simulink model "threshold_estimator"  (R2021a)
settings: Solver=FixedStepDiscrete  StartTime=0.0  StopTime=7.93555  RelTol=1e-3
undefined symbols (not defined in the file): lambda2
settings Model: DataTypeOverride=Off  Creator=Bhea Vasquez  LastModifiedBy=Bhea Vasquez
settings OptimizationCC: BlockReduction=off  ConditionallyExecuteInputs=off  DefaultParameterBehavior=Inlined
settings DebuggingCC: AlgebraicLoopMsg=error  SingleTaskRateTransMsg=error
settings HardwareCC: ProdBitPerPointer=32  ProdBitPerSizeT=32  ProdBitPerPtrDiffT=32  ProdLargestAtomicFloat=None  ProdIntDivRoundTo=Undefined  ProdEndianess=Unspecified  ProdWordSize=32  ProdHWDeviceType=ASIC/FPGA->ASIC/FPGA  TargetBitPerPointer=64  TargetBitPerSizeT=64  TargetBitPerPtrDiffT=64  TargetLongLongMode=on  TargetIntDivRoundTo=Zero  TargetEndianess=LittleEndian  TargetWordSize=64  TargetHWDeviceType=Custom Processor->MATLAB Host Computer  ProdEqTarget=off

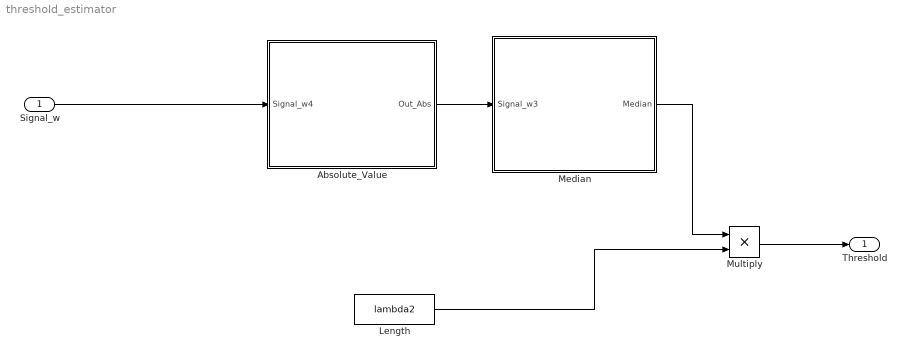
== system threshold_estimator ==
  Signal_w : Inport  OutDataTypeStr=fixdt(1,16,12)
  Absolute_Value : Subsystem
  Length : Constant  Value=lambda2  OutDataTypeStr=fixdt(1,16,12)  SampleTime=-1
  Median : Subsystem
  Multiply : Product  OutDataTypeStr=fixdt(1,16,12)  LockScale=on
  Threshold : Outport  OutDataTypeStr=fixdt(1,16,12)  VectorParamsAs1DForOutWhenUnconnected=off
  wires:
  Absolute_Value/1(Out_Abs) -> Median/1(Signal_w3)
  Signal_w/1 -> Absolute_Value/1(Signal_w4)
  Length/1 -> Multiply/2
  Multiply/1 -> Threshold/1
  Median/1(Median) -> Multiply/1

== system threshold_estimator/Absolute_Value ==
  Signal_w4 : Inport  OutDataTypeStr=fixdt(1,16,12)
  Absolute_Switch : Switch  Threshold=1  OutDataTypeStr=fixdt(1,16,12)
  Constant295 : Constant  Value=0  OutDataTypeStr=fixdt(1,16,12)  SampleTime=-1
  Gain2 : Gain  Gain=-1  ParamDataTypeStr=fixdt(1,16,12)  OutMin=-1  OutMax=-0.99  OutDataTypeStr=fixdt(1,16,12)
  Relational Operator2 : RelationalOperator  Operator=<  OutDataTypeStr=fixdt(1,16,12)  RndMeth=Simplest
  Out_Abs : Outport  OutDataTypeStr=fixdt(1,16,12)  VectorParamsAs1DForOutWhenUnconnected=off
  wires:
  Absolute_Switch/1 -> Out_Abs/1
  Relational Operator2/1 -> Absolute_Switch/2
  Gain2/1 -> Absolute_Switch/1
  Signal_w4/1 -> Absolute_Switch/3, Relational Operator2/1, Gain2/1
  Constant295/1 -> Relational Operator2/2

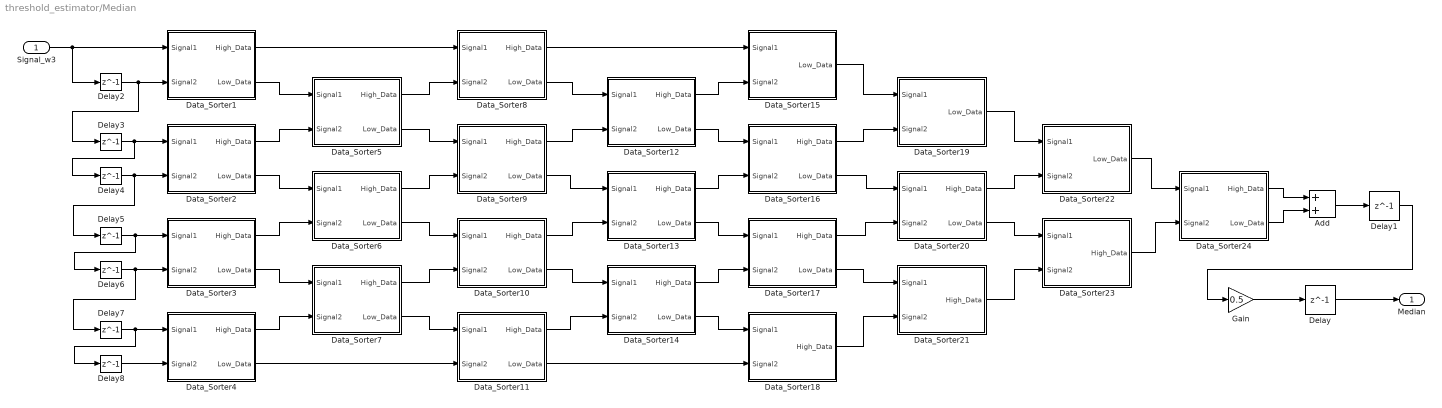
== system threshold_estimator/Median ==
  Signal_w3 : Inport  OutDataTypeStr=fixdt(1,16,12)
  Add : Sum  AccumDataTypeStr=fixdt(1,16,12)  OutDataTypeStr=fixdt(1,16,12)  LockScale=on
  Data_Sorter1 : Subsystem
  Data_Sorter10 : Subsystem
  Data_Sorter11 : Subsystem
  Data_Sorter12 : Subsystem
  Data_Sorter13 : Subsystem
  Data_Sorter14 : Subsystem
  Data_Sorter15 : Subsystem
  Data_Sorter16 : Subsystem
  Data_Sorter17 : Subsystem
  Data_Sorter18 : Subsystem
  Data_Sorter19 : Subsystem
  Data_Sorter2 : Subsystem
  Data_Sorter20 : Subsystem
  Data_Sorter21 : Subsystem
  Data_Sorter22 : Subsystem
  Data_Sorter23 : Subsystem
  Data_Sorter24 : Subsystem
  Data_Sorter3 : Subsystem
  Data_Sorter4 : Subsystem
  Data_Sorter5 : Subsystem
  Data_Sorter6 : Subsystem
  Data_Sorter7 : Subsystem
  Data_Sorter8 : Subsystem
  Data_Sorter9 : Subsystem
  Delay{,1..8} (9 alike) : Delay  DelayLength=1
  Gain : Gain  Gain=0.5  ParamDataTypeStr=fixdt(1,16,12)  OutMin=0.499  OutMax=0.5  OutDataTypeStr=fixdt(1,16,12)
  Median : Outport  OutDataTypeStr=fixdt(1,16,12)  VectorParamsAs1DForOutWhenUnconnected=off
  wires:
  Data_Sorter4/1(High_Data) -> Data_Sorter7/2(Signal2)
  Delay3/1 -> Delay4/1, Data_Sorter2/1(Signal1)
  Signal_w3/1 -> Data_Sorter1/1(Signal1), Delay2/1
  Data_Sorter10/1(High_Data) -> Data_Sorter13/2(Signal2)
  Data_Sorter23/1(High_Data) -> Data_Sorter24/2(Signal2)
  Data_Sorter12/2(Low_Data) -> Data_Sorter16/1(Signal1)
  Delay2/1 -> Delay3/1, Data_Sorter1/2(Signal2)
  Data_Sorter5/1(High_Data) -> Data_Sorter8/2(Signal2)
  Delay/1 -> Median/1
  Data_Sorter15/1(Low_Data) -> Data_Sorter19/1(Signal1)
  Add/1 -> Delay1/1
  Data_Sorter7/2(Low_Data) -> Data_Sorter11/1(Signal1)
  Data_Sorter24/1(High_Data) -> Add/1
  Data_Sorter1/2(Low_Data) -> Data_Sorter5/1(Signal1)
  Data_Sorter3/1(High_Data) -> Data_Sorter6/2(Signal2)
  Data_Sorter22/1(Low_Data) -> Data_Sorter24/1(Signal1)
  Data_Sorter2/1(High_Data) -> Data_Sorter5/2(Signal2)
  Data_Sorter10/2(Low_Data) -> Data_Sorter14/1(Signal1)
  Delay1/1 -> Gain/1
  Data_Sorter17/2(Low_Data) -> Data_Sorter21/1(Signal1)
  Data_Sorter21/1(High_Data) -> Data_Sorter23/2(Signal2)
  Data_Sorter7/1(High_Data) -> Data_Sorter10/2(Signal2)
  Delay4/1 -> Delay5/1, Data_Sorter2/2(Signal2)
  Data_Sorter16/1(High_Data) -> Data_Sorter19/2(Signal2)
  Data_Sorter20/1(High_Data) -> Data_Sorter22/2(Signal2)
  Data_Sorter16/2(Low_Data) -> Data_Sorter20/1(Signal1)
  Data_Sorter3/2(Low_Data) -> Data_Sorter7/1(Signal1)
  Data_Sorter2/2(Low_Data) -> Data_Sorter6/1(Signal1)
  Data_Sorter6/2(Low_Data) -> Data_Sorter10/1(Signal1)
  Data_Sorter19/1(Low_Data) -> Data_Sorter22/1(Signal1)
  Data_Sorter12/1(High_Data) -> Data_Sorter15/2(Signal2)
  Data_Sorter5/2(Low_Data) -> Data_Sorter9/1(Signal1)
  Data_Sorter24/2(Low_Data) -> Add/2
  Data_Sorter17/1(High_Data) -> Data_Sorter20/2(Signal2)
  Data_Sorter13/1(High_Data) -> Data_Sorter16/2(Signal2)
  Data_Sorter11/1(High_Data) -> Data_Sorter14/2(Signal2)
  Delay8/1 -> Data_Sorter4/2(Signal2)
  Data_Sorter8/2(Low_Data) -> Data_Sorter12/1(Signal1)
  Delay6/1 -> Delay7/1, Data_Sorter3/2(Signal2)
  Data_Sorter9/2(Low_Data) -> Data_Sorter13/1(Signal1)
  Data_Sorter4/2(Low_Data) -> Data_Sorter11/2(Signal2)
  Data_Sorter9/1(High_Data) -> Data_Sorter12/2(Signal2)
  Data_Sorter14/2(Low_Data) -> Data_Sorter18/1(Signal1)
  Delay5/1 -> Delay6/1, Data_Sorter3/1(Signal1)
  Delay7/1 -> Delay8/1, Data_Sorter4/1(Signal1)
  Data_Sorter1/1(High_Data) -> Data_Sorter8/1(Signal1)
  Data_Sorter8/1(High_Data) -> Data_Sorter15/1(Signal1)
  Data_Sorter14/1(High_Data) -> Data_Sorter17/2(Signal2)
  Data_Sorter6/1(High_Data) -> Data_Sorter9/2(Signal2)
  Data_Sorter20/2(Low_Data) -> Data_Sorter23/1(Signal1)
  Data_Sorter11/2(Low_Data) -> Data_Sorter18/2(Signal2)
  Data_Sorter13/2(Low_Data) -> Data_Sorter17/1(Signal1)
  Gain/1 -> Delay/1
  Data_Sorter18/1(High_Data) -> Data_Sorter21/2(Signal2)

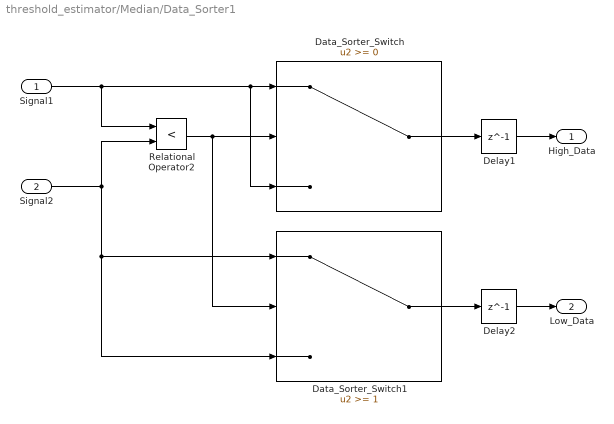
== system threshold_estimator/Median/Data_Sorter1 ==
  Signal1 : Inport  OutDataTypeStr=fixdt(1,16,12)
  Signal2 : Inport  Port=2  OutDataTypeStr=fixdt(1,16,12)
  Data_Sorter_Switch : Switch  OutDataTypeStr=fixdt(1,16,12)
  Data_Sorter_Switch1 : Switch  Threshold=1  OutDataTypeStr=fixdt(1,16,12)
  Delay1 : Delay  DelayLength=1
  Delay2 : Delay  DelayLength=1
  Relational Operator2 : RelationalOperator  Operator=<  OutDataTypeStr=fixdt(1,16,12)  RndMeth=Simplest
  High_Data : Outport  OutDataTypeStr=fixdt(1,16,12)  VectorParamsAs1DForOutWhenUnconnected=off
  Low_Data : Outport  Port=2  OutDataTypeStr=fixdt(1,16,12)  VectorParamsAs1DForOutWhenUnconnected=off
  wires:
  Signal1/1 -> Data_Sorter_Switch/3, Data_Sorter_Switch/1, Relational Operator2/1
  Relational Operator2/1 -> Data_Sorter_Switch1/2, Data_Sorter_Switch/2
  Signal2/1 -> Data_Sorter_Switch1/1, Data_Sorter_Switch1/3, Relational Operator2/2
  Data_Sorter_Switch1/1 -> Delay2/1
  Delay2/1 -> Low_Data/1
  Data_Sorter_Switch/1 -> Delay1/1
  Delay1/1 -> High_Data/1

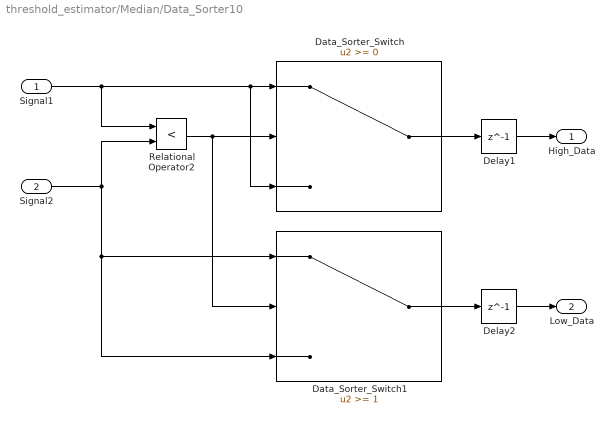
== system threshold_estimator/Median/Data_Sorter10 ==
  Signal1 : Inport  OutDataTypeStr=fixdt(1,16,12)
  Signal2 : Inport  Port=2  OutDataTypeStr=fixdt(1,16,12)
  Data_Sorter_Switch : Switch  OutDataTypeStr=fixdt(1,16,12)
  Data_Sorter_Switch1 : Switch  Threshold=1  OutDataTypeStr=fixdt(1,16,12)
  Delay1 : Delay  DelayLength=1
  Delay2 : Delay  DelayLength=1
  Relational Operator2 : RelationalOperator  Operator=<  OutDataTypeStr=fixdt(1,16,12)  RndMeth=Simplest
  High_Data : Outport  OutDataTypeStr=fixdt(1,16,12)  VectorParamsAs1DForOutWhenUnconnected=off
  Low_Data : Outport  Port=2  OutDataTypeStr=fixdt(1,16,12)  VectorParamsAs1DForOutWhenUnconnected=off
  wires:
  Signal1/1 -> Data_Sorter_Switch/3, Data_Sorter_Switch/1, Relational Operator2/1
  Relational Operator2/1 -> Data_Sorter_Switch1/2, Data_Sorter_Switch/2
  Signal2/1 -> Data_Sorter_Switch1/1, Data_Sorter_Switch1/3, Relational Operator2/2
  Data_Sorter_Switch1/1 -> Delay2/1
  Delay2/1 -> Low_Data/1
  Data_Sorter_Switch/1 -> Delay1/1
  Delay1/1 -> High_Data/1

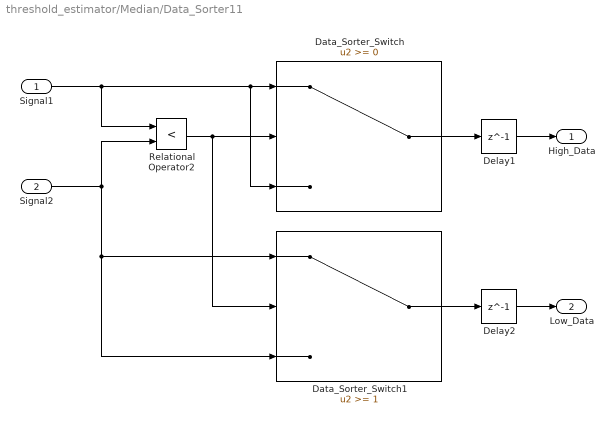
== system threshold_estimator/Median/Data_Sorter11 ==
  Signal1 : Inport  OutDataTypeStr=fixdt(1,16,12)
  Signal2 : Inport  Port=2  OutDataTypeStr=fixdt(1,16,12)
  Data_Sorter_Switch : Switch  OutDataTypeStr=fixdt(1,16,12)
  Data_Sorter_Switch1 : Switch  Threshold=1  OutDataTypeStr=fixdt(1,16,12)
  Delay1 : Delay  DelayLength=1
  Delay2 : Delay  DelayLength=1
  Relational Operator2 : RelationalOperator  Operator=<  OutDataTypeStr=fixdt(1,16,12)  RndMeth=Simplest
  High_Data : Outport  OutDataTypeStr=fixdt(1,16,12)  VectorParamsAs1DForOutWhenUnconnected=off
  Low_Data : Outport  Port=2  OutDataTypeStr=fixdt(1,16,12)  VectorParamsAs1DForOutWhenUnconnected=off
  wires:
  Signal1/1 -> Data_Sorter_Switch/3, Data_Sorter_Switch/1, Relational Operator2/1
  Relational Operator2/1 -> Data_Sorter_Switch1/2, Data_Sorter_Switch/2
  Signal2/1 -> Data_Sorter_Switch1/1, Data_Sorter_Switch1/3, Relational Operator2/2
  Data_Sorter_Switch1/1 -> Delay2/1
  Delay2/1 -> Low_Data/1
  Data_Sorter_Switch/1 -> Delay1/1
  Delay1/1 -> High_Data/1

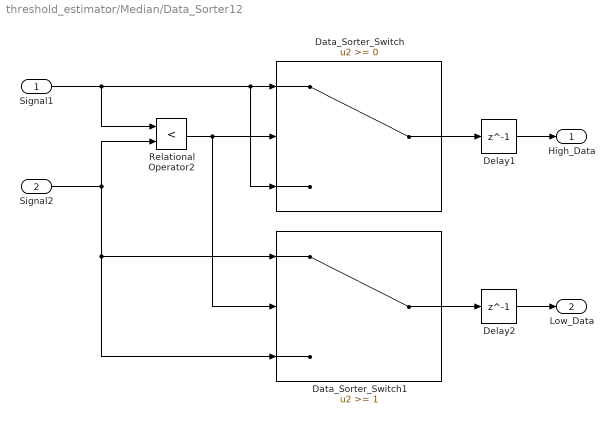
== system threshold_estimator/Median/Data_Sorter12 ==
  Signal1 : Inport  OutDataTypeStr=fixdt(1,16,12)
  Signal2 : Inport  Port=2  OutDataTypeStr=fixdt(1,16,12)
  Data_Sorter_Switch : Switch  OutDataTypeStr=fixdt(1,16,12)
  Data_Sorter_Switch1 : Switch  Threshold=1  OutDataTypeStr=fixdt(1,16,12)
  Delay1 : Delay  DelayLength=1
  Delay2 : Delay  DelayLength=1
  Relational Operator2 : RelationalOperator  Operator=<  OutDataTypeStr=fixdt(1,16,12)  RndMeth=Simplest
  High_Data : Outport  OutDataTypeStr=fixdt(1,16,12)  VectorParamsAs1DForOutWhenUnconnected=off
  Low_Data : Outport  Port=2  OutDataTypeStr=fixdt(1,16,12)  VectorParamsAs1DForOutWhenUnconnected=off
  wires:
  Signal1/1 -> Data_Sorter_Switch/3, Data_Sorter_Switch/1, Relational Operator2/1
  Relational Operator2/1 -> Data_Sorter_Switch1/2, Data_Sorter_Switch/2
  Signal2/1 -> Data_Sorter_Switch1/1, Data_Sorter_Switch1/3, Relational Operator2/2
  Data_Sorter_Switch1/1 -> Delay2/1
  Delay2/1 -> Low_Data/1
  Data_Sorter_Switch/1 -> Delay1/1
  Delay1/1 -> High_Data/1

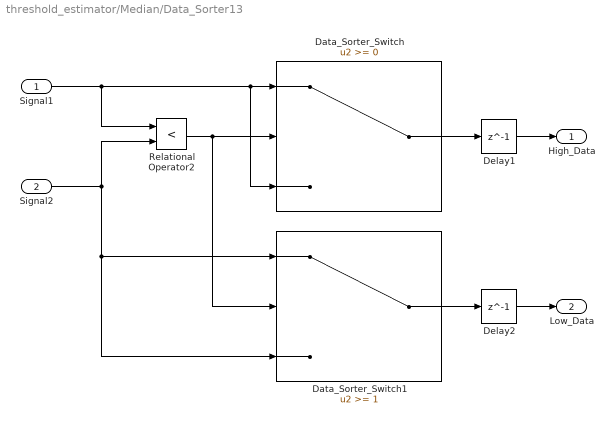
== system threshold_estimator/Median/Data_Sorter13 ==
  Signal1 : Inport  OutDataTypeStr=fixdt(1,16,12)
  Signal2 : Inport  Port=2  OutDataTypeStr=fixdt(1,16,12)
  Data_Sorter_Switch : Switch  OutDataTypeStr=fixdt(1,16,12)
  Data_Sorter_Switch1 : Switch  Threshold=1  OutDataTypeStr=fixdt(1,16,12)
  Delay1 : Delay  DelayLength=1
  Delay2 : Delay  DelayLength=1
  Relational Operator2 : RelationalOperator  Operator=<  OutDataTypeStr=fixdt(1,16,12)  RndMeth=Simplest
  High_Data : Outport  OutDataTypeStr=fixdt(1,16,12)  VectorParamsAs1DForOutWhenUnconnected=off
  Low_Data : Outport  Port=2  OutDataTypeStr=fixdt(1,16,12)  VectorParamsAs1DForOutWhenUnconnected=off
  wires:
  Signal1/1 -> Data_Sorter_Switch/3, Data_Sorter_Switch/1, Relational Operator2/1
  Relational Operator2/1 -> Data_Sorter_Switch1/2, Data_Sorter_Switch/2
  Signal2/1 -> Data_Sorter_Switch1/1, Data_Sorter_Switch1/3, Relational Operator2/2
  Data_Sorter_Switch1/1 -> Delay2/1
  Delay2/1 -> Low_Data/1
  Data_Sorter_Switch/1 -> Delay1/1
  Delay1/1 -> High_Data/1

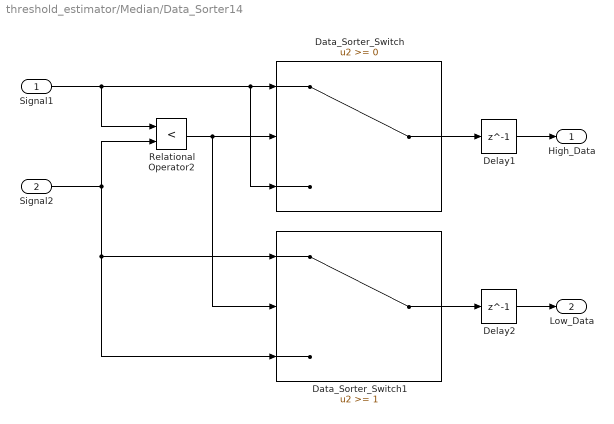
== system threshold_estimator/Median/Data_Sorter14 ==
  Signal1 : Inport  OutDataTypeStr=fixdt(1,16,12)
  Signal2 : Inport  Port=2  OutDataTypeStr=fixdt(1,16,12)
  Data_Sorter_Switch : Switch  OutDataTypeStr=fixdt(1,16,12)
  Data_Sorter_Switch1 : Switch  Threshold=1  OutDataTypeStr=fixdt(1,16,12)
  Delay1 : Delay  DelayLength=1
  Delay2 : Delay  DelayLength=1
  Relational Operator2 : RelationalOperator  Operator=<  OutDataTypeStr=fixdt(1,16,12)  RndMeth=Simplest
  High_Data : Outport  OutDataTypeStr=fixdt(1,16,12)  VectorParamsAs1DForOutWhenUnconnected=off
  Low_Data : Outport  Port=2  OutDataTypeStr=fixdt(1,16,12)  VectorParamsAs1DForOutWhenUnconnected=off
  wires:
  Signal1/1 -> Data_Sorter_Switch/3, Data_Sorter_Switch/1, Relational Operator2/1
  Relational Operator2/1 -> Data_Sorter_Switch1/2, Data_Sorter_Switch/2
  Signal2/1 -> Data_Sorter_Switch1/1, Data_Sorter_Switch1/3, Relational Operator2/2
  Data_Sorter_Switch1/1 -> Delay2/1
  Delay2/1 -> Low_Data/1
  Data_Sorter_Switch/1 -> Delay1/1
  Delay1/1 -> High_Data/1

== system threshold_estimator/Median/Data_Sorter15 ==
  Signal1 : Inport  OutDataTypeStr=fixdt(1,16,12)
  Signal2 : Inport  Port=2  OutDataTypeStr=fixdt(1,16,12)
  Data_Sorter_Switch1 : Switch  Threshold=1  OutDataTypeStr=fixdt(1,16,12)
  Delay2 : Delay  DelayLength=1
  Relational Operator2 : RelationalOperator  Operator=<  OutDataTypeStr=fixdt(1,16,12)  RndMeth=Simplest
  Low_Data : Outport  OutDataTypeStr=fixdt(1,16,12)  VectorParamsAs1DForOutWhenUnconnected=off
  wires:
  Signal1/1 -> Relational Operator2/1
  Relational Operator2/1 -> Data_Sorter_Switch1/2
  Signal2/1 -> Data_Sorter_Switch1/1, Data_Sorter_Switch1/3, Relational Operator2/2
  Data_Sorter_Switch1/1 -> Delay2/1
  Delay2/1 -> Low_Data/1

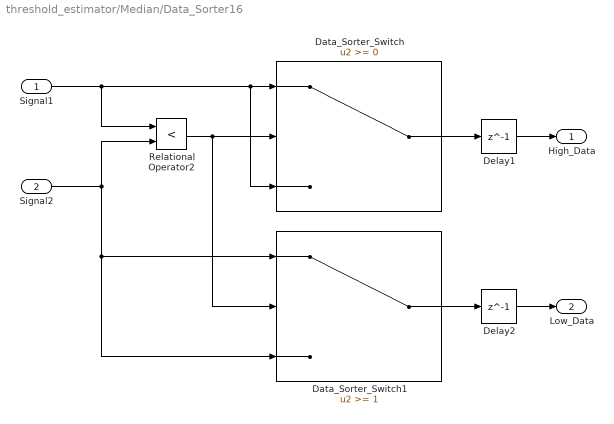
== system threshold_estimator/Median/Data_Sorter16 ==
  Signal1 : Inport  OutDataTypeStr=fixdt(1,16,12)
  Signal2 : Inport  Port=2  OutDataTypeStr=fixdt(1,16,12)
  Data_Sorter_Switch : Switch  OutDataTypeStr=fixdt(1,16,12)
  Data_Sorter_Switch1 : Switch  Threshold=1  OutDataTypeStr=fixdt(1,16,12)
  Delay1 : Delay  DelayLength=1
  Delay2 : Delay  DelayLength=1
  Relational Operator2 : RelationalOperator  Operator=<  OutDataTypeStr=fixdt(1,16,12)  RndMeth=Simplest
  High_Data : Outport  OutDataTypeStr=fixdt(1,16,12)  VectorParamsAs1DForOutWhenUnconnected=off
  Low_Data : Outport  Port=2  OutDataTypeStr=fixdt(1,16,12)  VectorParamsAs1DForOutWhenUnconnected=off
  wires:
  Signal1/1 -> Data_Sorter_Switch/3, Data_Sorter_Switch/1, Relational Operator2/1
  Relational Operator2/1 -> Data_Sorter_Switch1/2, Data_Sorter_Switch/2
  Signal2/1 -> Data_Sorter_Switch1/1, Data_Sorter_Switch1/3, Relational Operator2/2
  Data_Sorter_Switch1/1 -> Delay2/1
  Delay2/1 -> Low_Data/1
  Data_Sorter_Switch/1 -> Delay1/1
  Delay1/1 -> High_Data/1

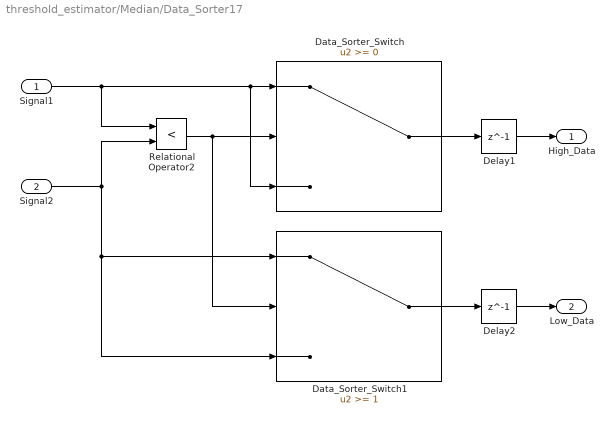
== system threshold_estimator/Median/Data_Sorter17 ==
  Signal1 : Inport  OutDataTypeStr=fixdt(1,16,12)
  Signal2 : Inport  Port=2  OutDataTypeStr=fixdt(1,16,12)
  Data_Sorter_Switch : Switch  OutDataTypeStr=fixdt(1,16,12)
  Data_Sorter_Switch1 : Switch  Threshold=1  OutDataTypeStr=fixdt(1,16,12)
  Delay1 : Delay  DelayLength=1
  Delay2 : Delay  DelayLength=1
  Relational Operator2 : RelationalOperator  Operator=<  OutDataTypeStr=fixdt(1,16,12)  RndMeth=Simplest
  High_Data : Outport  OutDataTypeStr=fixdt(1,16,12)  VectorParamsAs1DForOutWhenUnconnected=off
  Low_Data : Outport  Port=2  OutDataTypeStr=fixdt(1,16,12)  VectorParamsAs1DForOutWhenUnconnected=off
  wires:
  Signal1/1 -> Data_Sorter_Switch/3, Data_Sorter_Switch/1, Relational Operator2/1
  Relational Operator2/1 -> Data_Sorter_Switch1/2, Data_Sorter_Switch/2
  Signal2/1 -> Data_Sorter_Switch1/1, Data_Sorter_Switch1/3, Relational Operator2/2
  Data_Sorter_Switch1/1 -> Delay2/1
  Delay2/1 -> Low_Data/1
  Data_Sorter_Switch/1 -> Delay1/1
  Delay1/1 -> High_Data/1

== system threshold_estimator/Median/Data_Sorter18 ==
  Signal1 : Inport  OutDataTypeStr=fixdt(1,16,12)
  Signal2 : Inport  Port=2  OutDataTypeStr=fixdt(1,16,12)
  Data_Sorter_Switch1 : Switch  Threshold=1  OutDataTypeStr=fixdt(1,16,12)
  Delay2 : Delay  DelayLength=1
  Relational Operator2 : RelationalOperator  Operator=<  OutDataTypeStr=fixdt(1,16,12)  RndMeth=Simplest
  High_Data : Outport  OutDataTypeStr=fixdt(1,16,12)  VectorParamsAs1DForOutWhenUnconnected=off
  wires:
  Signal1/1 -> Relational Operator2/1
  Relational Operator2/1 -> Data_Sorter_Switch1/2
  Signal2/1 -> Data_Sorter_Switch1/1, Data_Sorter_Switch1/3, Relational Operator2/2
  Data_Sorter_Switch1/1 -> Delay2/1
  Delay2/1 -> High_Data/1

== system threshold_estimator/Median/Data_Sorter19 ==
  Signal1 : Inport  OutDataTypeStr=fixdt(1,16,12)
  Signal2 : Inport  Port=2  OutDataTypeStr=fixdt(1,16,12)
  Data_Sorter_Switch1 : Switch  Threshold=1  OutDataTypeStr=fixdt(1,16,12)
  Delay2 : Delay  DelayLength=1
  Relational Operator2 : RelationalOperator  Operator=<  OutDataTypeStr=fixdt(1,16,12)  RndMeth=Simplest
  Low_Data : Outport  OutDataTypeStr=fixdt(1,16,12)  VectorParamsAs1DForOutWhenUnconnected=off
  wires:
  Signal1/1 -> Relational Operator2/1
  Relational Operator2/1 -> Data_Sorter_Switch1/2
  Signal2/1 -> Data_Sorter_Switch1/1, Data_Sorter_Switch1/3, Relational Operator2/2
  Data_Sorter_Switch1/1 -> Delay2/1
  Delay2/1 -> Low_Data/1

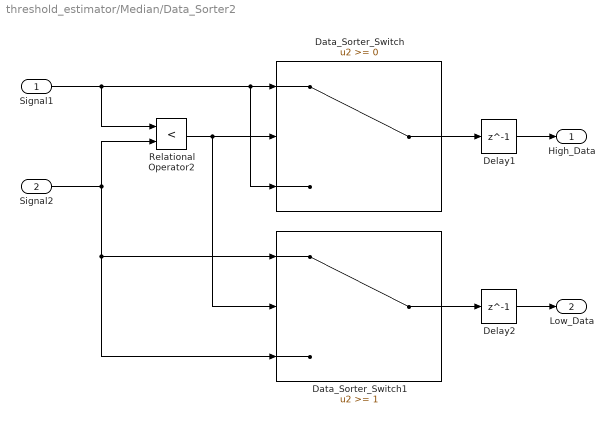
== system threshold_estimator/Median/Data_Sorter2 ==
  Signal1 : Inport  OutDataTypeStr=fixdt(1,16,12)
  Signal2 : Inport  Port=2  OutDataTypeStr=fixdt(1,16,12)
  Data_Sorter_Switch : Switch  OutDataTypeStr=fixdt(1,16,12)
  Data_Sorter_Switch1 : Switch  Threshold=1  OutDataTypeStr=fixdt(1,16,12)
  Delay1 : Delay  DelayLength=1
  Delay2 : Delay  DelayLength=1
  Relational Operator2 : RelationalOperator  Operator=<  OutDataTypeStr=fixdt(1,16,12)  RndMeth=Simplest
  High_Data : Outport  OutDataTypeStr=fixdt(1,16,12)  VectorParamsAs1DForOutWhenUnconnected=off
  Low_Data : Outport  Port=2  OutDataTypeStr=fixdt(1,16,12)  VectorParamsAs1DForOutWhenUnconnected=off
  wires:
  Signal1/1 -> Data_Sorter_Switch/3, Data_Sorter_Switch/1, Relational Operator2/1
  Relational Operator2/1 -> Data_Sorter_Switch1/2, Data_Sorter_Switch/2
  Signal2/1 -> Data_Sorter_Switch1/1, Data_Sorter_Switch1/3, Relational Operator2/2
  Data_Sorter_Switch1/1 -> Delay2/1
  Delay2/1 -> Low_Data/1
  Data_Sorter_Switch/1 -> Delay1/1
  Delay1/1 -> High_Data/1

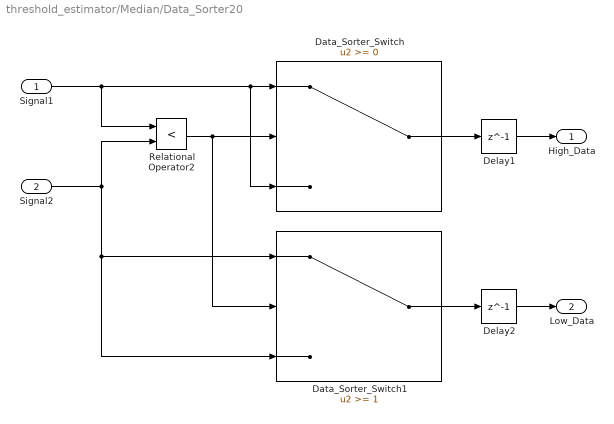
== system threshold_estimator/Median/Data_Sorter20 ==
  Signal1 : Inport  OutDataTypeStr=fixdt(1,16,12)
  Signal2 : Inport  Port=2  OutDataTypeStr=fixdt(1,16,12)
  Data_Sorter_Switch : Switch  OutDataTypeStr=fixdt(1,16,12)
  Data_Sorter_Switch1 : Switch  Threshold=1  OutDataTypeStr=fixdt(1,16,12)
  Delay1 : Delay  DelayLength=1
  Delay2 : Delay  DelayLength=1
  Relational Operator2 : RelationalOperator  Operator=<  OutDataTypeStr=fixdt(1,16,12)  RndMeth=Simplest
  High_Data : Outport  OutDataTypeStr=fixdt(1,16,12)  VectorParamsAs1DForOutWhenUnconnected=off
  Low_Data : Outport  Port=2  OutDataTypeStr=fixdt(1,16,12)  VectorParamsAs1DForOutWhenUnconnected=off
  wires:
  Signal1/1 -> Data_Sorter_Switch/3, Data_Sorter_Switch/1, Relational Operator2/1
  Relational Operator2/1 -> Data_Sorter_Switch1/2, Data_Sorter_Switch/2
  Signal2/1 -> Data_Sorter_Switch1/1, Data_Sorter_Switch1/3, Relational Operator2/2
  Data_Sorter_Switch1/1 -> Delay2/1
  Delay2/1 -> Low_Data/1
  Data_Sorter_Switch/1 -> Delay1/1
  Delay1/1 -> High_Data/1

== system threshold_estimator/Median/Data_Sorter21 ==
  Signal1 : Inport  OutDataTypeStr=fixdt(1,16,12)
  Signal2 : Inport  Port=2  OutDataTypeStr=fixdt(1,16,12)
  Data_Sorter_Switch1 : Switch  Threshold=1  OutDataTypeStr=fixdt(1,16,12)
  Delay2 : Delay  DelayLength=1
  Relational Operator2 : RelationalOperator  Operator=<  OutDataTypeStr=fixdt(1,16,12)  RndMeth=Simplest
  High_Data : Outport  OutDataTypeStr=fixdt(1,16,12)  VectorParamsAs1DForOutWhenUnconnected=off
  wires:
  Signal1/1 -> Relational Operator2/1
  Relational Operator2/1 -> Data_Sorter_Switch1/2
  Signal2/1 -> Data_Sorter_Switch1/1, Data_Sorter_Switch1/3, Relational Operator2/2
  Data_Sorter_Switch1/1 -> Delay2/1
  Delay2/1 -> High_Data/1

== system threshold_estimator/Median/Data_Sorter22 ==
  Signal1 : Inport  OutDataTypeStr=fixdt(1,16,12)
  Signal2 : Inport  Port=2  OutDataTypeStr=fixdt(1,16,12)
  Data_Sorter_Switch1 : Switch  Threshold=1  OutDataTypeStr=fixdt(1,16,12)
  Delay2 : Delay  DelayLength=1
  Relational Operator2 : RelationalOperator  Operator=<  OutDataTypeStr=fixdt(1,16,12)  RndMeth=Simplest
  Low_Data : Outport  OutDataTypeStr=fixdt(1,16,12)  VectorParamsAs1DForOutWhenUnconnected=off
  wires:
  Signal1/1 -> Relational Operator2/1
  Relational Operator2/1 -> Data_Sorter_Switch1/2
  Signal2/1 -> Data_Sorter_Switch1/1, Data_Sorter_Switch1/3, Relational Operator2/2
  Data_Sorter_Switch1/1 -> Delay2/1
  Delay2/1 -> Low_Data/1

== system threshold_estimator/Median/Data_Sorter23 ==
  Signal1 : Inport  OutDataTypeStr=fixdt(1,16,12)
  Signal2 : Inport  Port=2  OutDataTypeStr=fixdt(1,16,12)
  Data_Sorter_Switch1 : Switch  Threshold=1  OutDataTypeStr=fixdt(1,16,12)
  Delay2 : Delay  DelayLength=1
  Relational Operator2 : RelationalOperator  Operator=<  OutDataTypeStr=fixdt(1,16,12)  RndMeth=Simplest
  High_Data : Outport  OutDataTypeStr=fixdt(1,16,12)  VectorParamsAs1DForOutWhenUnconnected=off
  wires:
  Signal1/1 -> Relational Operator2/1
  Relational Operator2/1 -> Data_Sorter_Switch1/2
  Signal2/1 -> Data_Sorter_Switch1/1, Data_Sorter_Switch1/3, Relational Operator2/2
  Data_Sorter_Switch1/1 -> Delay2/1
  Delay2/1 -> High_Data/1

== system threshold_estimator/Median/Data_Sorter24 ==
  Signal1 : Inport  OutDataTypeStr=fixdt(1,16,12)
  Signal2 : Inport  Port=2  OutDataTypeStr=fixdt(1,16,12)
  Data_Sorter_Switch : Switch  OutDataTypeStr=fixdt(1,16,12)
  Data_Sorter_Switch1 : Switch  Threshold=1  OutDataTypeStr=fixdt(1,16,12)
  Delay1 : Delay  DelayLength=1
  Delay2 : Delay  DelayLength=1
  Relational Operator2 : RelationalOperator  Operator=<  OutDataTypeStr=fixdt(1,16,12)  RndMeth=Simplest
  High_Data : Outport  OutDataTypeStr=fixdt(1,16,12)  VectorParamsAs1DForOutWhenUnconnected=off
  Low_Data : Outport  Port=2  OutDataTypeStr=fixdt(1,16,12)  VectorParamsAs1DForOutWhenUnconnected=off
  wires:
  Signal1/1 -> Data_Sorter_Switch/3, Data_Sorter_Switch/1, Relational Operator2/1
  Relational Operator2/1 -> Data_Sorter_Switch1/2, Data_Sorter_Switch/2
  Signal2/1 -> Data_Sorter_Switch1/1, Data_Sorter_Switch1/3, Relational Operator2/2
  Data_Sorter_Switch1/1 -> Delay2/1
  Delay2/1 -> Low_Data/1
  Data_Sorter_Switch/1 -> Delay1/1
  Delay1/1 -> High_Data/1

== system threshold_estimator/Median/Data_Sorter3 ==
  Signal1 : Inport  OutDataTypeStr=fixdt(1,16,12)
  Signal2 : Inport  Port=2  OutDataTypeStr=fixdt(1,16,12)
  Data_Sorter_Switch : Switch  OutDataTypeStr=fixdt(1,16,12)
  Data_Sorter_Switch1 : Switch  Threshold=1  OutDataTypeStr=fixdt(1,16,12)
  Delay1 : Delay  DelayLength=1
  Delay2 : Delay  DelayLength=1
  Relational Operator2 : RelationalOperator  Operator=<  OutDataTypeStr=fixdt(1,16,12)  RndMeth=Simplest
  High_Data : Outport  OutDataTypeStr=fixdt(1,16,12)  VectorParamsAs1DForOutWhenUnconnected=off
  Low_Data : Outport  Port=2  OutDataTypeStr=fixdt(1,16,12)  VectorParamsAs1DForOutWhenUnconnected=off
  wires:
  Signal1/1 -> Data_Sorter_Switch/3, Data_Sorter_Switch/1, Relational Operator2/1
  Relational Operator2/1 -> Data_Sorter_Switch1/2, Data_Sorter_Switch/2
  Signal2/1 -> Data_Sorter_Switch1/1, Data_Sorter_Switch1/3, Relational Operator2/2
  Data_Sorter_Switch1/1 -> Delay2/1
  Delay2/1 -> Low_Data/1
  Data_Sorter_Switch/1 -> Delay1/1
  Delay1/1 -> High_Data/1

== system threshold_estimator/Median/Data_Sorter4 ==
  Signal1 : Inport  OutDataTypeStr=fixdt(1,16,12)
  Signal2 : Inport  Port=2  OutDataTypeStr=fixdt(1,16,12)
  Data_Sorter_Switch : Switch  OutDataTypeStr=fixdt(1,16,12)
  Data_Sorter_Switch1 : Switch  Threshold=1  OutDataTypeStr=fixdt(1,16,12)
  Delay1 : Delay  DelayLength=1
  Delay2 : Delay  DelayLength=1
  Relational Operator2 : RelationalOperator  Operator=<  OutDataTypeStr=fixdt(1,16,12)  RndMeth=Simplest
  High_Data : Outport  OutDataTypeStr=fixdt(1,16,12)  VectorParamsAs1DForOutWhenUnconnected=off
  Low_Data : Outport  Port=2  OutDataTypeStr=fixdt(1,16,12)  VectorParamsAs1DForOutWhenUnconnected=off
  wires:
  Signal1/1 -> Data_Sorter_Switch/3, Data_Sorter_Switch/1, Relational Operator2/1
  Relational Operator2/1 -> Data_Sorter_Switch1/2, Data_Sorter_Switch/2
  Signal2/1 -> Data_Sorter_Switch1/1, Data_Sorter_Switch1/3, Relational Operator2/2
  Data_Sorter_Switch1/1 -> Delay2/1
  Delay2/1 -> Low_Data/1
  Data_Sorter_Switch/1 -> Delay1/1
  Delay1/1 -> High_Data/1

== system threshold_estimator/Median/Data_Sorter5 ==
  Signal1 : Inport  OutDataTypeStr=fixdt(1,16,12)
  Signal2 : Inport  Port=2  OutDataTypeStr=fixdt(1,16,12)
  Data_Sorter_Switch : Switch  OutDataTypeStr=fixdt(1,16,12)
  Data_Sorter_Switch1 : Switch  Threshold=1  OutDataTypeStr=fixdt(1,16,12)
  Delay1 : Delay  DelayLength=1
  Delay2 : Delay  DelayLength=1
  Relational Operator2 : RelationalOperator  Operator=<  OutDataTypeStr=fixdt(1,16,12)  RndMeth=Simplest
  High_Data : Outport  OutDataTypeStr=fixdt(1,16,12)  VectorParamsAs1DForOutWhenUnconnected=off
  Low_Data : Outport  Port=2  OutDataTypeStr=fixdt(1,16,12)  VectorParamsAs1DForOutWhenUnconnected=off
  wires:
  Signal1/1 -> Data_Sorter_Switch/3, Data_Sorter_Switch/1, Relational Operator2/1
  Relational Operator2/1 -> Data_Sorter_Switch1/2, Data_Sorter_Switch/2
  Signal2/1 -> Data_Sorter_Switch1/1, Data_Sorter_Switch1/3, Relational Operator2/2
  Data_Sorter_Switch1/1 -> Delay2/1
  Delay2/1 -> Low_Data/1
  Data_Sorter_Switch/1 -> Delay1/1
  Delay1/1 -> High_Data/1

== system threshold_estimator/Median/Data_Sorter6 ==
  Signal1 : Inport  OutDataTypeStr=fixdt(1,16,12)
  Signal2 : Inport  Port=2  OutDataTypeStr=fixdt(1,16,12)
  Data_Sorter_Switch : Switch  OutDataTypeStr=fixdt(1,16,12)
  Data_Sorter_Switch1 : Switch  Threshold=1  OutDataTypeStr=fixdt(1,16,12)
  Delay1 : Delay  DelayLength=1
  Delay2 : Delay  DelayLength=1
  Relational Operator2 : RelationalOperator  Operator=<  OutDataTypeStr=fixdt(1,16,12)  RndMeth=Simplest
  High_Data : Outport  OutDataTypeStr=fixdt(1,16,12)  VectorParamsAs1DForOutWhenUnconnected=off
  Low_Data : Outport  Port=2  OutDataTypeStr=fixdt(1,16,12)  VectorParamsAs1DForOutWhenUnconnected=off
  wires:
  Signal1/1 -> Data_Sorter_Switch/3, Data_Sorter_Switch/1, Relational Operator2/1
  Relational Operator2/1 -> Data_Sorter_Switch1/2, Data_Sorter_Switch/2
  Signal2/1 -> Data_Sorter_Switch1/1, Data_Sorter_Switch1/3, Relational Operator2/2
  Data_Sorter_Switch1/1 -> Delay2/1
  Delay2/1 -> Low_Data/1
  Data_Sorter_Switch/1 -> Delay1/1
  Delay1/1 -> High_Data/1

== system threshold_estimator/Median/Data_Sorter7 ==
  Signal1 : Inport  OutDataTypeStr=fixdt(1,16,12)
  Signal2 : Inport  Port=2  OutDataTypeStr=fixdt(1,16,12)
  Data_Sorter_Switch : Switch  OutDataTypeStr=fixdt(1,16,12)
  Data_Sorter_Switch1 : Switch  Threshold=1  OutDataTypeStr=fixdt(1,16,12)
  Delay1 : Delay  DelayLength=1
  Delay2 : Delay  DelayLength=1
  Relational Operator2 : RelationalOperator  Operator=<  OutDataTypeStr=fixdt(1,16,12)  RndMeth=Simplest
  High_Data : Outport  OutDataTypeStr=fixdt(1,16,12)  VectorParamsAs1DForOutWhenUnconnected=off
  Low_Data : Outport  Port=2  OutDataTypeStr=fixdt(1,16,12)  VectorParamsAs1DForOutWhenUnconnected=off
  wires:
  Signal1/1 -> Data_Sorter_Switch/3, Data_Sorter_Switch/1, Relational Operator2/1
  Relational Operator2/1 -> Data_Sorter_Switch1/2, Data_Sorter_Switch/2
  Signal2/1 -> Data_Sorter_Switch1/1, Data_Sorter_Switch1/3, Relational Operator2/2
  Data_Sorter_Switch1/1 -> Delay2/1
  Delay2/1 -> Low_Data/1
  Data_Sorter_Switch/1 -> Delay1/1
  Delay1/1 -> High_Data/1

== system threshold_estimator/Median/Data_Sorter8 ==
  Signal1 : Inport  OutDataTypeStr=fixdt(1,16,12)
  Signal2 : Inport  Port=2  OutDataTypeStr=fixdt(1,16,12)
  Data_Sorter_Switch : Switch  OutDataTypeStr=fixdt(1,16,12)
  Data_Sorter_Switch1 : Switch  Threshold=1  OutDataTypeStr=fixdt(1,16,12)
  Delay1 : Delay  DelayLength=1
  Delay2 : Delay  DelayLength=1
  Relational Operator2 : RelationalOperator  Operator=<  OutDataTypeStr=fixdt(1,16,12)  RndMeth=Simplest
  High_Data : Outport  OutDataTypeStr=fixdt(1,16,12)  VectorParamsAs1DForOutWhenUnconnected=off
  Low_Data : Outport  Port=2  OutDataTypeStr=fixdt(1,16,12)  VectorParamsAs1DForOutWhenUnconnected=off
  wires:
  Signal1/1 -> Data_Sorter_Switch/3, Data_Sorter_Switch/1, Relational Operator2/1
  Relational Operator2/1 -> Data_Sorter_Switch1/2, Data_Sorter_Switch/2
  Signal2/1 -> Data_Sorter_Switch1/1, Data_Sorter_Switch1/3, Relational Operator2/2
  Data_Sorter_Switch1/1 -> Delay2/1
  Delay2/1 -> Low_Data/1
  Data_Sorter_Switch/1 -> Delay1/1
  Delay1/1 -> High_Data/1

== system threshold_estimator/Median/Data_Sorter9 ==
  Signal1 : Inport  OutDataTypeStr=fixdt(1,16,12)
  Signal2 : Inport  Port=2  OutDataTypeStr=fixdt(1,16,12)
  Data_Sorter_Switch : Switch  OutDataTypeStr=fixdt(1,16,12)
  Data_Sorter_Switch1 : Switch  Threshold=1  OutDataTypeStr=fixdt(1,16,12)
  Delay1 : Delay  DelayLength=1
  Delay2 : Delay  DelayLength=1
  Relational Operator2 : RelationalOperator  Operator=<  OutDataTypeStr=fixdt(1,16,12)  RndMeth=Simplest
  High_Data : Outport  OutDataTypeStr=fixdt(1,16,12)  VectorParamsAs1DForOutWhenUnconnected=off
  Low_Data : Outport  Port=2  OutDataTypeStr=fixdt(1,16,12)  VectorParamsAs1DForOutWhenUnconnected=off
  wires:
  Signal1/1 -> Data_Sorter_Switch/3, Data_Sorter_Switch/1, Relational Operator2/1
  Relational Operator2/1 -> Data_Sorter_Switch1/2, Data_Sorter_Switch/2
  Signal2/1 -> Data_Sorter_Switch1/1, Data_Sorter_Switch1/3, Relational Operator2/2
  Data_Sorter_Switch1/1 -> Delay2/1
  Delay2/1 -> Low_Data/1
  Data_Sorter_Switch/1 -> Delay1/1
  Delay1/1 -> High_Data/1
